simulink model "yolov8SimulinkSupport"  (R2024b)
settings: Solver=VariableStepAuto  StartTime=0.0  StopTime=1  RelTol=1e-3
libraries: visionsources x1
settings Model: Creator=viakkala  LastModifiedBy=viakkala
settings SolverCC: DateTimeAtSimulationTimeZero=[]
settings SFSimCC: SimTargetLang=C++

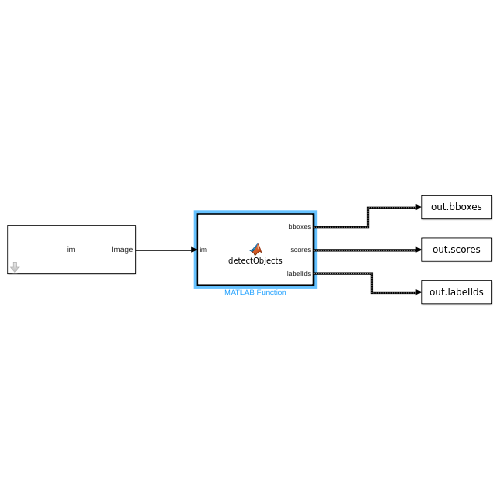
[thumbnail: Simulink's stored preview of the top-level diagram]
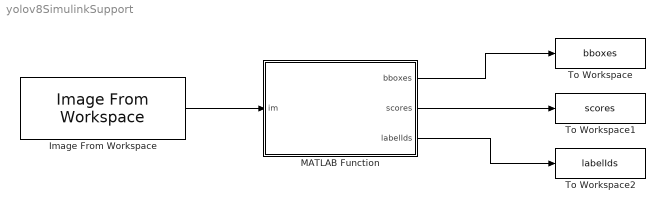
== system yolov8SimulinkSupport ==
  Image From Workspace : visionsources/Image From Workspace  Tag=vipblks_nd  ImageValue=im  Ts=1  imagePorts=One multidimensional signal  OutPortLabels=R|G|B  ImageDataType=Inherit from 'Value'  Signed=on  WordLength=16  sdImageDataType=sfix(16)  FractionLengthMode=User-defined  FractionLength=15
  MATLAB Function : MATLAB Function  TreatAsAtomicUnit=on
  To Workspace : ToWorkspace  VariableName=bboxes  SaveFormat=Timeseries  SampleTime=1
  To Workspace1 : ToWorkspace  VariableName=scores  SaveFormat=Timeseries  SampleTime=1
  To Workspace2 : ToWorkspace  VariableName=labelIds  SaveFormat=Timeseries  SampleTime=1
  wires:
  Image From Workspace/1 -> MATLAB Function/1(im)
  MATLAB Function/1(bboxes) -> To Workspace/1
  MATLAB Function/2(scores) -> To Workspace1/1
  MATLAB Function/3(labelIds) -> To Workspace2/1

== matlab function yolov8SimulinkSupport/MATLAB Function ==
  data: im input; bboxes output size=[10 4]; scores output size=10; labelIds output size=10
function [bboxes,scores,labelIds]  = detectObjects(im)

%codegen
coder.varsize('class_name',[1 100]);
persistent det

if isempty(det)
    det = coder.loadDeepLearningNetwork('yolov8n.mat');
end

% origSize = size(im);
% newSize = size(im);
% 
% % Convert uint8 to single
% I = single(im);
% 
% % Rescale image pixes to [0,1]
% Iout = I./255;

% Get the input size of the network.
inputSize = [640 640 3];

% Apply Preprocessing on the input image.
origSize = size(im);
Ibgr = im(:,:,[3,2,1]); % convert image to bgr
img = helper.preprocess(Ibgr, inputSize);

newSize = size(img);
Iout = img(:,:,[3,2,1]); % convert image to rgb

dlInput = dlarray(Iout, 'SSCB');

numClasses = 80;
outFeatureMaps = cell(3,1);
[outFeatureMaps{:}] = predict(det, dlInput);

% Apply postprocessing on the output feature maps.
[bboxes,scores,labelIds] = helper.postprocess(outFeatureMaps, ...
    origSize, newSize, numClasses);

end
